simulink model "rad_selection"  (R2024b)
settings: Solver=VariableStepAuto  StartTime=0.0  StopTime=720  RelTol=1e-3
values from neighbouring files (symbols this model uses):
  ali_rad_W = 0.017    [Custom_Script.m]
  efficiencyGrid = min(efficiencyGrid, 0.96)    [Custom_Script.m]    (also in EmraxEfficiencyMap.m)
  speed = linspace(min(eff_rpm), max(eff_rpm), 100)    [Custom_Script.m]    (also in EmraxEfficiencyMap.m = linspace(min(rpm), max(rpm), 100))
  torque = linspace(min(torque), max(torque), 100)    [EmraxEfficiencyMap.m]    (also in load_emrax_map.m = data{:, 2})
undefined symbols (not defined in the file or in its folder): ali_air_area_flow, crf_air_area_flow, current_air_area_flow, mishi_air_area_flow, mishi_rad_W
libraries: fl_lib x35, nesl_utility x16, SimscapeFluids_lib x7
(part 2 of 2)

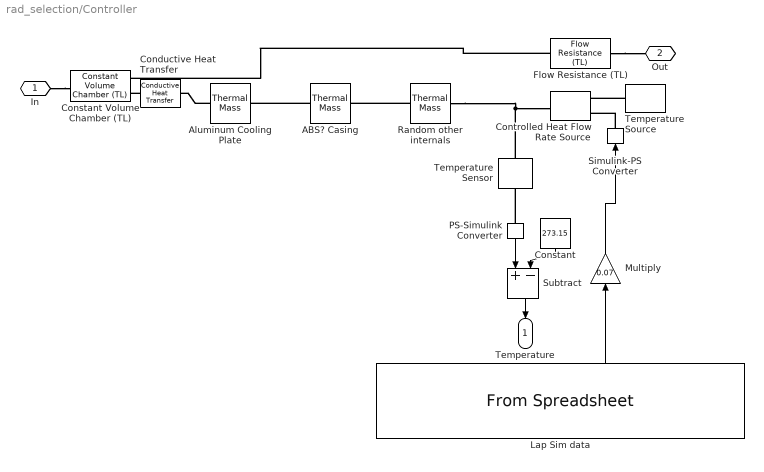
== system rad_selection/Controller ==
  ABS? Casing : fl_lib/Thermal/Thermal Elements/Thermal Mass  mass_type=foundation.enum.constant_variable.constant  mass=1 kg  sp_heat=1500 J/(K*kg)  mass_min=1e-6 kg  num_ports=foundation.enum.numPorts2.two  m_specify=off  m_priority=High  m=1 kg  m_nominal_specify=off  m_nominal_value=1  m_nominal_unit=kg  T_specify=on  T_priority=High  T=35 degC  T_nominal_specify=off  T_nominal_value=1  T_nominal_unit=K  Q_specify=off  Q_priority=None  Q=0 W  Q_nominal_specify=off  Q_nominal_value=1  Q_nominal_unit=W
      settings: InternalSimscapePortConfiguration="{\"Bottom\":[],\"Left\":[{\"id\":\"M\",\"label\":\"\",\"type\":\"foundation.thermal.thermal\"}],\"Right\":[{\"id\":\"N\",\"label\":\"\",\"type\":\"foundation.thermal.thermal\"}],\"Top\":[]}"
  Aluminum Cooling Plate : fl_lib/Thermal/Thermal Elements/Thermal Mass  mass_type=foundation.enum.constant_variable.constant  mass=2 kg  sp_heat=903 J/(K*kg)  mass_min=1e-6 kg  num_ports=foundation.enum.numPorts2.two  m_specify=off  m_priority=High  m=1 kg  m_nominal_specify=off  m_nominal_value=1  m_nominal_unit=kg  T_specify=on  T_priority=High  T=35 degC  T_nominal_specify=off  T_nominal_value=1  T_nominal_unit=K  Q_specify=off  Q_priority=None  Q=0 W  Q_nominal_specify=off  Q_nominal_value=1  Q_nominal_unit=W
      settings: InternalSimscapePortConfiguration="{\"Bottom\":[],\"Left\":[{\"id\":\"M\",\"label\":\"\",\"type\":\"foundation.thermal.thermal\"}],\"Right\":[{\"id\":\"N\",\"label\":\"\",\"type\":\"foundation.thermal.thermal\"}],\"Top\":[]}"
  Conductive Heat Transfer : fl_lib/Thermal/Thermal Elements/Conductive Heat Transfer  thermal_type=foundation.enum.ConstantVariableTabulated.Constant  wall_geometry=foundation.enum.ConductionWallGeometry.Planar  area=200*230 mm^2  thickness=10 mm  d_in=0.05 m  d_out=0.1 m  L=1 m  th_cond_min=10 W/(K*m)  th_cond=237 W/(K*m)  th_cond_TLU=[413, 401, 392, 383, 371, 357, 342] W/(K*m)  temp_TLU=[200, 273, 400, 600, 800, 1000, 1200] K  T_specify=off  T_priority=None  T=0 K  T_nominal_specify=off  T_nominal_value=1  T_nominal_unit=K  Q_specify=off  Q_priority=None  Q=0 W  Q_nominal_specify=off  Q_nominal_value=1  Q_nominal_unit=W
  Constant : Constant  Value=273.15
  Constant Volume Chamber (TL) : fl_lib/Thermal Liquid/Elements/Constant Volume Chamber (TL)  volume=0.1 l  num_ports=foundation.enum.num_ports.two  area_A=0.01 m^2  area_B=0.01 m^2  area_C=0.01 m^2  area_D=0.01 m^2  p_I_specify=off  p_I_priority=High  p_I=0.101325 MPa  p_I_nominal_specify=off  p_I_nominal_value=1  p_I_nominal_unit=MPa  T_I_specify=on  T_I_priority=High  T_I=35 degC  T_I_nominal_specify=off  T_I_nominal_value=1  T_I_nominal_unit=K  u_I_specify=off  u_I_priority=None  u_I=83.906 kJ/kg  u_I_nominal_specify=off  u_I_nominal_value=1  u_I_nominal_unit=kJ/kg  rho_I_specify=off  rho_I_priority=None  rho_I=998.21 kg/m^3  rho_I_nominal_specify=off  rho_I_nominal_value=1  rho_I_nominal_unit=kg/m^3
      settings: InternalSimscapePortConfiguration="{\"Bottom\":[],\"Left\":[{\"id\":\"A\",\"label\":\"A\",\"type\":\"foundation.thermal_liquid.thermal_liquid\"},{\"id\":\"H\",\"label\":\"H\",\"type\":\"foundation.thermal.thermal\"}],\"Right\":[{\"id\":\"B\",\"label\":\"B\",\"type\":\"foundation.thermal_liquid.thermal_liquid\"}],\"Top\":[]}"
  Controlled Heat Flow Rate Source : fl_lib/Thermal/Thermal Sources/Controlled Heat Flow Rate Source
  Flow Resistance (TL) : fl_lib/Thermal Liquid/Elements/Flow Resistance (TL)  delta_p_nominal=0.56 bar  mdot_nominal=0.17 kg/s  area=0.01 m^2  laminar_fraction=1e-3
  Lap Sim data : FromSpreadsheet  FileName=C:\Users\noahk\School\UCalgary Racing\2024-25\Projects\UCR02-CoolingSim\data\LapTime_Power_new__10.xlsx  SheetName=LapTime_Power_new__10  SampleTime=0.1
  Multiply : Gain  Gain=0.07
  PS-Simulink Converter : nesl_utility/PS-Simulink Converter  PhysicalDomain=network_engine_domain  SubClassName=ps_output  LeftPortType=input  RightPortType=output  PseudoPeriodic=off  Frequencies=[]  VectorFormat=inherit  Unit=inherit  AffineConversion=off
  Random other internals : fl_lib/Thermal/Thermal Elements/Thermal Mass  mass_type=foundation.enum.constant_variable.constant  mass=7 kg  sp_heat=500 J/(K*kg)  mass_min=1e-6 kg  num_ports=foundation.enum.numPorts2.two  m_specify=off  m_priority=High  m=1 kg  m_nominal_specify=off  m_nominal_value=1  m_nominal_unit=kg  T_specify=on  T_priority=High  T=35 degC  T_nominal_specify=off  T_nominal_value=1  T_nominal_unit=K  Q_specify=off  Q_priority=None  Q=0 W  Q_nominal_specify=off  Q_nominal_value=1  Q_nominal_unit=W
      settings: InternalSimscapePortConfiguration="{\"Bottom\":[],\"Left\":[{\"id\":\"M\",\"label\":\"\",\"type\":\"foundation.thermal.thermal\"}],\"Right\":[{\"id\":\"N\",\"label\":\"\",\"type\":\"foundation.thermal.thermal\"}],\"Top\":[]}"
  Simulink-PS Converter : nesl_utility/Simulink-PS Converter  PhysicalDomain=network_engine_domain  SubClassName=ps_input  LeftPortType=input  RightPortType=output  PseudoPeriodic=off  Frequencies=[]  NoiseDistribution=none  NoiseParameters=[]  Unit=1  AffineConversion=off  FilteringAndDerivatives=provide  SimscapeFilterOrder=1  InputFilterTimeConstant=0.001  UdotUserProvided=0
  Subtract : Sum  Inputs=+-
  Temperature Sensor : fl_lib/Thermal/Thermal Sensors/Temperature Sensor  temperature_measure=foundation.enum.MeasurementReference.absolute
      settings: InternalSimscapePortConfiguration="{\"Bottom\":[],\"Left\":[{\"id\":\"A\",\"label\":\"A\",\"type\":\"foundation.thermal.thermal\"}],\"Right\":[{\"id\":\"T\",\"label\":\"T\",\"type\":\"output\"}],\"Top\":[]}"
  Temperature Source : fl_lib/Thermal/Thermal Sources/Temperature Source  temperature=35 degC
  In : PMIOPort  Side=Left
  Out : PMIOPort  Port=2  Side=Right
  Temperature : Outport
  wires:
  Lap Sim data/3 -> Multiply/1
  Multiply/1 -> Simulink-PS Converter/1
  Subtract/1 -> Temperature/1
  PS-Simulink Converter/1 -> Subtract/1
  Constant/1 -> Subtract/2
  connections:
  Flow Resistance (TL)/LConn1 -- Constant Volume Chamber (TL)/LConn1
  Simulink-PS Converter/RConn1 -- Controlled Heat Flow Rate Source/RConn1
  Flow Resistance (TL)/RConn1 -- Out/RConn1
  Temperature Source/LConn1 -- Controlled Heat Flow Rate Source/RConn2
  In/RConn1 -- Constant Volume Chamber (TL)/RConn1
  Temperature Sensor/LConn1 -- Random other internals/LConn1 -- Controlled Heat Flow Rate Source/LConn1
  PS-Simulink Converter/LConn1 -- Temperature Sensor/RConn1
  Conductive Heat Transfer/RConn1 -- Constant Volume Chamber (TL)/LConn2
  Aluminum Cooling Plate/RConn1 -- Conductive Heat Transfer/LConn1
  ABS? Casing/RConn1 -- Aluminum Cooling Plate/LConn1
  Random other internals/RConn1 -- ABS? Casing/LConn1

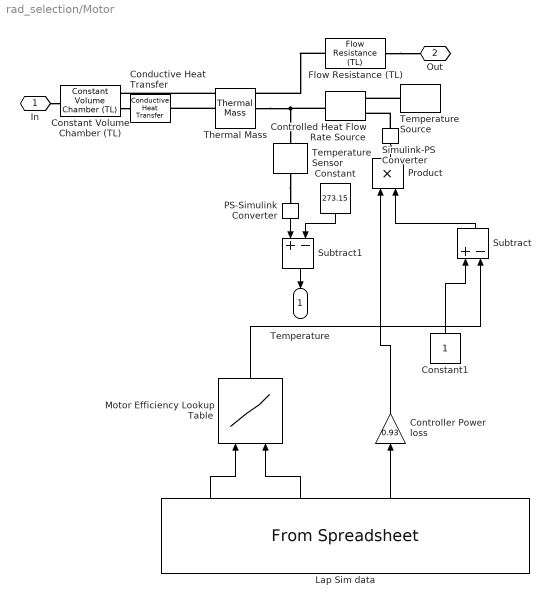
== system rad_selection/Motor ==
  Conductive Heat Transfer : fl_lib/Thermal/Thermal Elements/Conductive Heat Transfer  thermal_type=foundation.enum.ConstantVariableTabulated.Constant  wall_geometry=foundation.enum.ConductionWallGeometry.Cylindrical  area=100*100 mm^2  thickness=0.1 m  d_in=8 mm  d_out=10 mm  L=2 m  th_cond_min=10 W/(K*m)  th_cond=237 W/(K*m)  th_cond_TLU=[413, 401, 392, 383, 371, 357, 342] W/(K*m)  temp_TLU=[200, 273, 400, 600, 800, 1000, 1200] K  T_specify=off  T_priority=None  T=0 K  T_nominal_specify=off  T_nominal_value=1  T_nominal_unit=K  Q_specify=off  Q_priority=None  Q=0 W  Q_nominal_specify=off  Q_nominal_value=1  Q_nominal_unit=W
  Constant : Constant  Value=273.15
  Constant Volume Chamber (TL) : fl_lib/Thermal Liquid/Elements/Constant Volume Chamber (TL)  volume=1e-4 m^3  num_ports=foundation.enum.num_ports.two  area_A=0.01 m^2  area_B=0.01 m^2  area_C=0.01 m^2  area_D=0.01 m^2  p_I_specify=off  p_I_priority=High  p_I=0.101325 MPa  p_I_nominal_specify=off  p_I_nominal_value=1  p_I_nominal_unit=MPa  T_I_specify=on  T_I_priority=High  T_I=35 degC  T_I_nominal_specify=off  T_I_nominal_value=1  T_I_nominal_unit=K  u_I_specify=off  u_I_priority=None  u_I=83.906 kJ/kg  u_I_nominal_specify=off  u_I_nominal_value=1  u_I_nominal_unit=kJ/kg  rho_I_specify=off  rho_I_priority=None  rho_I=998.21 kg/m^3  rho_I_nominal_specify=off  rho_I_nominal_value=1  rho_I_nominal_unit=kg/m^3
      settings: InternalSimscapePortConfiguration="{\"Bottom\":[],\"Left\":[{\"id\":\"A\",\"label\":\"A\",\"type\":\"foundation.thermal_liquid.thermal_liquid\"},{\"id\":\"H\",\"label\":\"H\",\"type\":\"foundation.thermal.thermal\"}],\"Right\":[{\"id\":\"B\",\"label\":\"B\",\"type\":\"foundation.thermal_liquid.thermal_liquid\"}],\"Top\":[]}"
  Constant1 : Constant
  Controlled Heat Flow Rate Source : fl_lib/Thermal/Thermal Sources/Controlled Heat Flow Rate Source
  Controller Power loss : Gain  Gain=0.93
  Flow Resistance (TL) : fl_lib/Thermal Liquid/Elements/Flow Resistance (TL)  delta_p_nominal=0.5 bar  mdot_nominal=0.1 kg/s  area=0.01 m^2  laminar_fraction=1e-3
  Lap Sim data : FromSpreadsheet  FileName=C:\Users\noahk\School\UCalgary Racing\2024-25\Projects\UCR02-CoolingSim\data\LapTime_Power_new__10.xlsx  SheetName=LapTime_Power_new__10  SampleTime=0.1
  Motor Efficiency Lookup Table : Lookup_n-D  BreakpointsForDimension1=speed  BreakpointsForDimension2=torque  Table=efficiencyGrid  InternalRulePriority=Speed  RndMeth=Simplest
      settings: InputPortMap=u0,u1
  PS-Simulink Converter : nesl_utility/PS-Simulink Converter  PhysicalDomain=network_engine_domain  SubClassName=ps_output  LeftPortType=input  RightPortType=output  PseudoPeriodic=off  Frequencies=[]  VectorFormat=inherit  Unit=inherit  AffineConversion=off
  Product : Product
  Simulink-PS Converter : nesl_utility/Simulink-PS Converter  PhysicalDomain=network_engine_domain  SubClassName=ps_input  LeftPortType=input  RightPortType=output  PseudoPeriodic=off  Frequencies=[]  NoiseDistribution=none  NoiseParameters=[]  Unit=1  AffineConversion=off  FilteringAndDerivatives=provide  SimscapeFilterOrder=1  InputFilterTimeConstant=0.001  UdotUserProvided=0
  Subtract : Sum  Inputs=+-
  Subtract1 : Sum  Inputs=+-
  Temperature Sensor : fl_lib/Thermal/Thermal Sensors/Temperature Sensor  temperature_measure=foundation.enum.MeasurementReference.absolute
      settings: InternalSimscapePortConfiguration="{\"Bottom\":[],\"Left\":[{\"id\":\"A\",\"label\":\"A\",\"type\":\"foundation.thermal.thermal\"}],\"Right\":[{\"id\":\"T\",\"label\":\"T\",\"type\":\"output\"}],\"Top\":[]}"
  Temperature Source : fl_lib/Thermal/Thermal Sources/Temperature Source  temperature=35 degC
  Thermal Mass : fl_lib/Thermal/Thermal Elements/Thermal Mass  mass_type=foundation.enum.constant_variable.constant  mass=6 kg  sp_heat=903 J/(K*kg)  mass_min=1e-6 kg  num_ports=foundation.enum.numPorts2.two  m_specify=off  m_priority=High  m=1 kg  m_nominal_specify=off  m_nominal_value=1  m_nominal_unit=kg  T_specify=on  T_priority=High  T=35 degC  T_nominal_specify=off  T_nominal_value=1  T_nominal_unit=K  Q_specify=off  Q_priority=None  Q=0 W  Q_nominal_specify=off  Q_nominal_value=1  Q_nominal_unit=W
      settings: InternalSimscapePortConfiguration="{\"Bottom\":[],\"Left\":[{\"id\":\"M\",\"label\":\"\",\"type\":\"foundation.thermal.thermal\"}],\"Right\":[{\"id\":\"N\",\"label\":\"\",\"type\":\"foundation.thermal.thermal\"}],\"Top\":[]}"
  In : PMIOPort  Side=Left
  Out : PMIOPort  Port=2  Side=Right
  Temperature : Outport
  wires:
  Motor Efficiency Lookup Table/1 -> Subtract/2
  Constant1/1 -> Subtract/1
  Subtract/1 -> Product/2
  Product/1 -> Simulink-PS Converter/1
  Lap Sim data/1 -> Motor Efficiency Lookup Table/1
  Lap Sim data/2 -> Motor Efficiency Lookup Table/2
  Controller Power loss/1 -> Product/1
  Lap Sim data/3 -> Controller Power loss/1
  PS-Simulink Converter/1 -> Subtract1/1
  Constant/1 -> Subtract1/2
  Subtract1/1 -> Temperature/1
  connections:
  Simulink-PS Converter/RConn1 -- Controlled Heat Flow Rate Source/RConn1
  In/RConn1 -- Constant Volume Chamber (TL)/RConn1
  Temperature Source/LConn1 -- Controlled Heat Flow Rate Source/RConn2
  Flow Resistance (TL)/LConn1 -- Constant Volume Chamber (TL)/LConn1
  Flow Resistance (TL)/RConn1 -- Out/RConn1
  Temperature Sensor/RConn1 -- PS-Simulink Converter/LConn1
  Controlled Heat Flow Rate Source/LConn1 -- Temperature Sensor/LConn1 -- Thermal Mass/LConn1
  Constant Volume Chamber (TL)/LConn2 -- Conductive Heat Transfer/RConn1
  Thermal Mass/RConn1 -- Conductive Heat Transfer/LConn1
